simulink model "test_joystick"  (R2015b)
settings: Solver=FixedStepAuto  StartTime=0.0  StopTime=inf  FixedStep=0.1  RelTol=1e-3
libraries: simulink_extras x2, aerolibanimutils x1
settings Model: Creator=rcasado  LastModifiedBy=rcasado

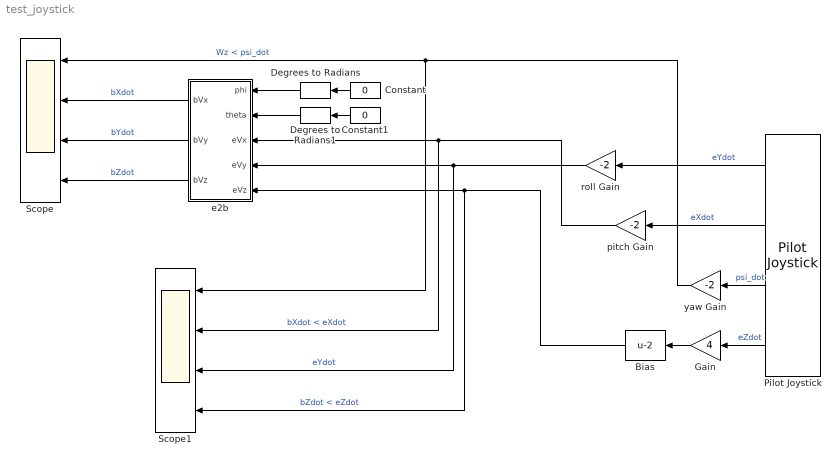
== system test_joystick ==
  Bias : Bias  Bias=-2
  Constant : Constant  Value=0
  Constant1 : Constant  Value=0
  Degrees to Radians : simulink_extras/Transformations/Degrees to Radians
  Degrees to Radians1 : simulink_extras/Transformations/Degrees to Radians
  Gain : Gain  Gain=4
  Pilot Joystick : aerolibanimutils/Pilot Joystick  JoystickID=Joystick1  OutputConfiguration=FourAxis  SampleTime=1/10
  Scope : Scope  NumInputPorts=4
  Scope1 : Scope  NumInputPorts=4
  e2b : Subsystem
  pitch Gain : Gain  Gain=-2
  roll Gain : Gain  Gain=-2
  yaw Gain : Gain  Gain=-2
  wires:
  e2b/3(bVz) -> Scope/4  "bZdot"
  e2b/1(bVx) -> Scope/2  "bXdot"
  e2b/2(bVy) -> Scope/3  "bYdot"
  Bias/1 -> Scope1/4, e2b/5(eVz)  "bZdot < eZdot"
  Pilot Joystick/4 -> Gain/1  "eZdot"
  roll Gain/1 -> Scope1/3, e2b/4(eVy)  "eYdot"
  Gain/1 -> Bias/1
  Pilot Joystick/3 -> yaw Gain/1  "psi_dot"
  Pilot Joystick/2 -> pitch Gain/1  "eXdot"
  Pilot Joystick/1 -> roll Gain/1  "eYdot"
  pitch Gain/1 -> Scope1/2, e2b/3(eVx)  "bXdot < eXdot"
  yaw Gain/1 -> Scope1/1, Scope/1  "Wz < psi_dot"
  Constant/1 -> Degrees to Radians/1
  Degrees to Radians/1 -> e2b/1(phi)
  Constant1/1 -> Degrees to Radians1/1
  Degrees to Radians1/1 -> e2b/2(theta)

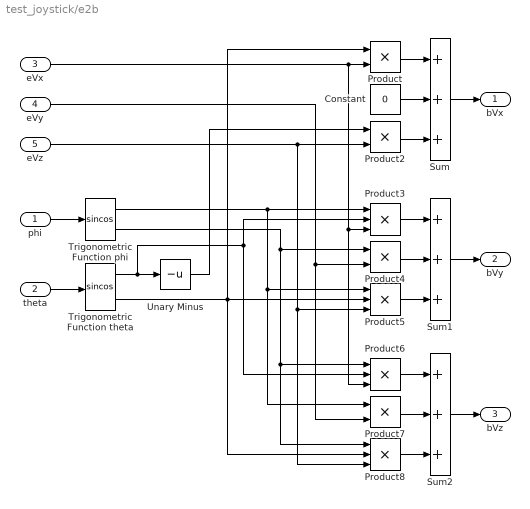
== system test_joystick/e2b ==
  phi : Inport
  theta : Inport  Port=2
  eVx : Inport  Port=3
  eVy : Inport  Port=4
  eVz : Inport  Port=5
  Constant : Constant  Value=0
  Product{,2,4,7} (4 alike) : Product
  Product{3,5..6,8} (4 alike) : Product  Inputs=3
  Sum : Sum  Inputs=3
  Sum1 : Sum  Inputs=3
  Sum2 : Sum  Inputs=3
  Trigonometric Function phi : Trigonometry  Operator=sincos
  Trigonometric Function theta : Trigonometry  Operator=sincos
  Unary Minus : UnaryMinus
  bVx : Outport
  bVy : Outport  Port=2
  bVz : Outport  Port=3
  wires:
  theta/1 -> Trigonometric Function theta/1
  phi/1 -> Trigonometric Function phi/1
  Trigonometric Function phi/2 -> Product8/1, Product6/1, Product4/1
  Trigonometric Function theta/2 -> Product/1, Product8/2, Product5/2
  Trigonometric Function theta/1 -> Product3/2, Product6/2, Unary Minus/1
  Trigonometric Function phi/1 -> Product5/1, Product7/1, Product3/1
  Sum/1 -> bVx/1
  Sum1/1 -> bVy/1
  Sum2/1 -> bVz/1
  Product/1 -> Sum/1
  Constant/1 -> Sum/2
  Product2/1 -> Sum/3
  Product3/1 -> Sum1/1
  Product4/1 -> Sum1/2
  Product5/1 -> Sum1/3
  Product6/1 -> Sum2/1
  Product7/1 -> Sum2/2
  Product8/1 -> Sum2/3
  eVx/1 -> Product6/3, Product3/3, Product/2
  eVy/1 -> Product7/2, Product4/2
  eVz/1 -> Product8/3, Product5/3, Product2/2
  Unary Minus/1 -> Product2/1
